simulink model "leg_2_4_simulink(another way)"  (R2019a)
settings: Solver=VariableStepAuto  StartTime=0.0  StopTime=20  RelTol=1e-3
values from neighbouring files (symbols this model uses):
  g = 9.81    [leg_1_6.m]    (also in leg_2_4_simulink(another way).m; leg_controller.m)
  Jm = 0.000506    [leg_2_4_simulink(another way).m]    (also in leg_controller.m)
  k = 20000    [leg_2_4_simulink(another way).m]    (also in leg_controller.m)
  Kd = 100    [leg_2_4_simulink(another way).m]    (also in leg_controller.m = 1000)
  Kd_s = 2    [leg_2_4_simulink(another way).m]    (also in leg_controller.m = 5)
  Ki = 7000    [leg_2_4_simulink(another way).m]    (also in leg_controller.m = 4500)
  Ki_s = 0.5    [leg_2_4_simulink(another way).m]    (also in leg_controller.m = 0)
  Kp = 16000    [leg_2_4_simulink(another way).m]    (also in leg_controller.m = 8000)
  Kp_s = 2    [leg_2_4_simulink(another way).m]    (also in leg_controller.m = 10)
  m = 80    [leg_2_4_simulink(another way).m]    (also in leg_controller.m)
  N = 40    [leg_2_4_simulink(another way).m]    (also in leg_controller.m)
  r = 0.05    [leg_2_4_simulink(another way).m]    (also in leg_controller.m)
  Tau_max = 1.313    [leg_2_4_simulink(another way).m]    (also in leg_controller.m)
  yo = 1    [leg_1_6.m]    (also in leg_2_4_simulink(another way).m; leg_controller.m)
undefined symbols (not defined in the file or in its folder): ydes
libraries: simulink x2
settings Model: Creator=apple  LastModifiedBy=apple
settings SolverCC: ZeroCrossAlgorithm=Adaptive
settings DataIOCC: SaveFormat=Array  ReturnWorkspaceOutputs=off
settings DebuggingCC: IgnoredZcDiagnostic=none

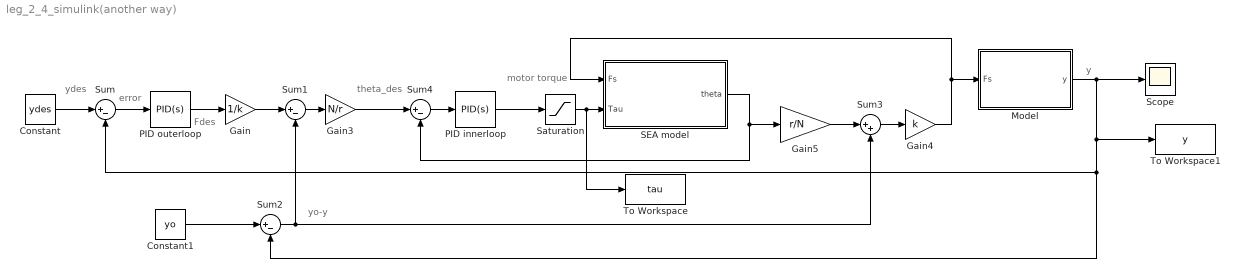
== system leg_2_4_simulink(another way) ==
  note: yo-y
  note: ydes
  note: y
  note: error
  note: Fdes
  note: motor
      | torque
  note: theta_des
  Constant : Constant  Value=ydes
  Constant1 : Constant  Value=yo
  Gain : Gain  Gain=1/k
  Gain3 : Gain  Gain=N/r
  Gain4 : Gain  Gain=k
  Gain5 : Gain  Gain=r/N
  Model : Subsystem
  PID innerloop : simulink/Continuous/PID Controller  Controller=PID  Form=Parallel  TimeDomain=Continuous-time  SampleTime=-1  IntegratorMethod=Forward Euler  FilterMethod=Forward Euler  ControllerParametersSource=internal  P=Kp_s  I=Ki_s  D=Kd_s  UseFilter=on  N=100  TunerSelectOption=Transfer Function Based (PID Tuner App)  InitialConditionSource=internal  InitialConditionForIntegrator=0  InitialConditionForFilter=0  DifferentiatorICPrevScaledInput=0  ExternalReset=none  TrackingMode=off  Kt=1  LimitOutput=off  UpperSaturationLimit=inf  LowerSaturationLimit=-inf  LinearizeAsGain=on  AntiWindupMode=none  Kb=1  POutMin=[]  POutMax=[]  IOutMin=[]  IOutMax=[]  DOutMin=[]  DOutMax=[]  NOutMin=[]  NOutMax=[]  SumOutMin=[]  SumOutMax=[]  SaturationOutMin=[]  SaturationOutMax=[]  PParamMin=[]  PParamMax=[]  IParamMin=[]  IParamMax=[]  DParamMin=[]  DParamMax=[]  NParamMin=[]  NParamMax=[]  KbParamMin=[]  KbParamMax=[]  KtParamMin=[]  KtParamMax=[]  KbOutMin=[]  KbOutMax=[]  KtOutMin=[]  KtOutMax=[]  IntegratorOutMin=[]  IntegratorOutMax=[]  FilterOutMin=[]  FilterOutMax=[]  SumI1OutMin=[]  SumI1OutMax=[]  SumI2OutMin=[]  SumI2OutMax=[]  SumI3OutMin=[]  SumI3OutMax=[]  SumI4OutMin=[]  SumI4OutMax=[]  SumDOutMin=[]  SumDOutMax=[]  DifferentiatorOutMin=[]  DifferentiatorOutMax=[]  FilterDiffOutCoefMin=[]  FilterDiffOutCoefMax=[]  ReciprocalOutMin=[]  ReciprocalOutMax=[]  SumDenOutMin=[]  SumDenOutMax=[]  SumNumOutMin=[]  SumNumOutMax=[]  DivideOutMin=[]  DivideOutMax=[]  IntegratorContinuousStateAttributes=''  IntegratorStateMustResolveToSignalObject=off  IntegratorRTWStateStorageClass=Auto  FilterContinuousStateAttributes=''  FilterStateMustResolveToSignalObject=off  FilterRTWStateStorageClass=Auto  ParallelPVariant=InternalParameters  IdealPVariant=Disabled  IVariant=InternalParameters  DVariant=InternalParameters  IntegratorVariant=Continuous  SatVariant=Disabled  AWVariant=Passthrough  PCopyVariant=Disabled  TRVariant=Disabled  FdbkBlocksVariant=Forward  IdealPFdbkVariant=Disabled  SatFdbkVariant=Disabled  DerivativeFilterVariant=ContFilter  NVariant=InternalParameters  NCopyVariant=Disabled  FilterICVariant=InternalICsFilter  IntegratorICVariant=InternalICs  ExternalResetVariant=Disabled  TRSumVariant=Passthrough  SumFdbkVariant=Disabled  SumVariant=Sum_PID
  PID outerloop : simulink/Continuous/PID Controller  Controller=PID  Form=Parallel  TimeDomain=Continuous-time  SampleTime=-1  IntegratorMethod=Forward Euler  FilterMethod=Forward Euler  ControllerParametersSource=internal  P=Kp  I=Ki  D=Kd  UseFilter=on  N=100  TunerSelectOption=Transfer Function Based (PID Tuner App)  InitialConditionSource=internal  InitialConditionForIntegrator=0  InitialConditionForFilter=0  DifferentiatorICPrevScaledInput=0  ExternalReset=none  TrackingMode=off  Kt=1  LimitOutput=off  UpperSaturationLimit=inf  LowerSaturationLimit=-inf  LinearizeAsGain=on  AntiWindupMode=none  Kb=1  POutMin=[]  POutMax=[]  IOutMin=[]  IOutMax=[]  DOutMin=[]  DOutMax=[]  NOutMin=[]  NOutMax=[]  SumOutMin=[]  SumOutMax=[]  SaturationOutMin=[]  SaturationOutMax=[]  PParamMin=[]  PParamMax=[]  IParamMin=[]  IParamMax=[]  DParamMin=[]  DParamMax=[]  NParamMin=[]  NParamMax=[]  KbParamMin=[]  KbParamMax=[]  KtParamMin=[]  KtParamMax=[]  KbOutMin=[]  KbOutMax=[]  KtOutMin=[]  KtOutMax=[]  IntegratorOutMin=[]  IntegratorOutMax=[]  FilterOutMin=[]  FilterOutMax=[]  SumI1OutMin=[]  SumI1OutMax=[]  SumI2OutMin=[]  SumI2OutMax=[]  SumI3OutMin=[]  SumI3OutMax=[]  SumI4OutMin=[]  SumI4OutMax=[]  SumDOutMin=[]  SumDOutMax=[]  DifferentiatorOutMin=[]  DifferentiatorOutMax=[]  FilterDiffOutCoefMin=[]  FilterDiffOutCoefMax=[]  ReciprocalOutMin=[]  ReciprocalOutMax=[]  SumDenOutMin=[]  SumDenOutMax=[]  SumNumOutMin=[]  SumNumOutMax=[]  DivideOutMin=[]  DivideOutMax=[]  IntegratorContinuousStateAttributes=''  IntegratorStateMustResolveToSignalObject=off  IntegratorRTWStateStorageClass=Auto  FilterContinuousStateAttributes=''  FilterStateMustResolveToSignalObject=off  FilterRTWStateStorageClass=Auto  ParallelPVariant=InternalParameters  IdealPVariant=Disabled  IVariant=InternalParameters  DVariant=InternalParameters  IntegratorVariant=Continuous  SatVariant=Disabled  AWVariant=Passthrough  PCopyVariant=Disabled  TRVariant=Disabled  FdbkBlocksVariant=Forward  IdealPFdbkVariant=Disabled  SatFdbkVariant=Disabled  DerivativeFilterVariant=ContFilter  NVariant=InternalParameters  NCopyVariant=Disabled  FilterICVariant=InternalICsFilter  IntegratorICVariant=InternalICs  ExternalResetVariant=Disabled  TRSumVariant=Passthrough  SumFdbkVariant=Disabled  SumVariant=Sum_PID
  SEA model : Subsystem
  Saturation : Saturate  UpperLimit=Tau_max  LowerLimit=-Tau_max
  Scope : Scope
  Sum{,1..2,4} (4 alike) : Sum  Inputs=|+-
  Sum3 : Sum  Inputs=|++
  To Workspace : ToWorkspace  VariableName=tau  SampleTime=-1
  To Workspace1 : ToWorkspace  VariableName=y  SampleTime=-1
  wires:
  Constant/1 -> Sum/1
  Sum1/1 -> Gain3/1
  Gain3/1 -> Sum4/1
  Sum3/1 -> Gain4/1
  Constant1/1 -> Sum2/1
  Sum2/1 -> Sum1/2, Sum3/2
  Gain4/1 -> Model/1(Fs), SEA model/1(Fs)
  Gain5/1 -> Sum3/1
  Gain/1 -> Sum1/1
  Sum/1 -> PID outerloop/1
  PID outerloop/1 -> Gain/1
  Sum4/1 -> PID innerloop/1
  PID innerloop/1 -> Saturation/1
  SEA model/1("theta ") -> Gain5/1, Sum4/2
  Saturation/1 -> To Workspace/1, SEA model/2(Tau)
  Model/1(y) -> Scope/1, To Workspace1/1, Sum2/2, Sum/2

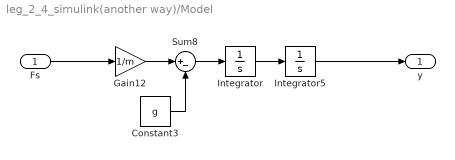
== system leg_2_4_simulink(another way)/Model ==
  Fs : Inport
  Constant3 : Constant  Value=g
  Gain12 : Gain  Gain=1/m
  Integrator : Integrator
  Integrator5 : Integrator  InitialCondition=1
  Sum8 : Sum  Inputs=|+-
  y : Outport
  wires:
  Fs/1 -> Gain12/1
  Integrator5/1 -> y/1
  Sum8/1 -> Integrator/1
  Integrator/1 -> Integrator5/1
  Constant3/1 -> Sum8/2
  Gain12/1 -> Sum8/1

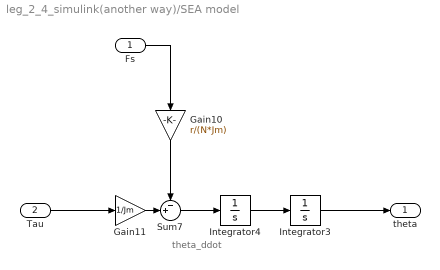
== system leg_2_4_simulink(another way)/SEA model ==
  note: theta_ddot
  Fs : Inport
  Tau : Inport  Port=2
  Gain10 : Gain  Gain=r/(N*Jm)
  Gain11 : Gain  Gain=1/Jm
  Integrator3 : Integrator
  Integrator4 : Integrator
  Sum7 : Sum  Inputs=-+|
  "theta " : Outport
  wires:
  Integrator3/1 -> "theta "/1
  Gain11/1 -> Sum7/2
  Tau/1 -> Gain11/1
  Fs/1 -> Gain10/1
  Integrator4/1 -> Integrator3/1
  Gain10/1 -> Sum7/1
  Sum7/1 -> Integrator4/1
